simulink model "q3"  (R2021a)
settings: Solver=VariableStepAuto  StartTime=0.0  StopTime=8*1e-6  RelTol=1e-3
libraries: commdigbbndpm3 x2, commrandsrc3 x1
settings Model: Creator=Fatiha  LastModifiedBy=Fatiha

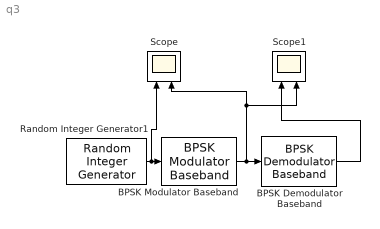
== system q3 ==
  BPSK Demodulator Baseband : commdigbbndpm3/BPSK Demodulator Baseband  DecType=Hard decision  VarSource=Dialog  Variance=1  Ph=0  outDtype=Inherit via internal rule  derotateFactorWordLen=16  derotateFactorDataTypeStr=Inherit: Same word length as input  derotateFactorLastDataTypeStr=Inherit: Same word length as input
  BPSK Modulator Baseband : commdigbbndpm3/BPSK Modulator Baseband  Ph=0  outDtype=double  outWordLen=16  outUDDataType=sfix(16)  outFracLenMode=Best precision  outFracLen=15  outDataTypeStr=double  outLastDataTypeStr=double
  Random Integer Generator1 : commrandsrc3/Random Integer Generator  SetSize=2  SeedSource=Auto  Seed=0  SampleTime=1e-6  SamplesPerFrame=1  OutputDataType=double  SimulateUsing=Interpreted execution
  Scope : Scope  NumInputPorts=2
  Scope1 : Scope  NumInputPorts=2
  wires:
  BPSK Demodulator Baseband/1 -> Scope1/1
  Random Integer Generator1/1 -> BPSK Modulator Baseband/1, Scope/1
  BPSK Modulator Baseband/1 -> BPSK Demodulator Baseband/1, Scope1/2, Scope/2
